simulink model "Controle_v_teta"  (R2018a)
settings: Solver=VariableStepAuto  StartTime=0.0  StopTime=5  RelTol=1e-3
values from neighbouring files (symbols this model uses):
  KDw = 4/(Kw*ts_w)    (= 3.21802091714)    [LineFollower.m]
  KIm = Pm*KPm    (= 0.759312111233)    [LineFollower.m]    (also in malha_fechada.m)
  Km = 455.5    [LineFollower.m]    (also in malha_aberta.m; malha_fechada.m)
  KPm = 4/(Km*ts_m)    (= 0.0585437248445)    [LineFollower.m]    (also in malha_fechada.m)
  KPw = Pw*KDw    (= 80.0965406275)    [LineFollower.m]
  l = 69e-3    (= 0.069)    [LineFollower.m]    (also in malha_aberta.m; malha_fechada.m)
  Pm = 12.97    [LineFollower.m]    (also in malha_aberta.m; malha_fechada.m)
  r = 16e-3    (= 0.016)    [LineFollower.m]    (also in kinematic_model.m; malha_aberta.m; malha_fechada.m)
undefined symbols (not defined in the file or in its folder): KIw
libraries: simulink x3
settings Model: Creator=bruno  LastModifiedBy=bruno

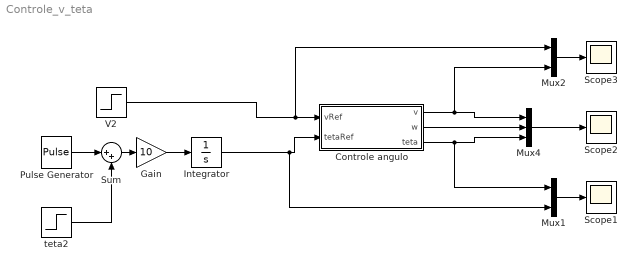
== system Controle_v_teta ==
  Controle angulo : Subsystem
  Gain : Gain  Gain=10
  Integrator : Integrator
  Mux1 : Mux  Inputs=2
  Mux2 : Mux  Inputs=2
  Mux4 : Mux  Inputs=3
  Pulse Generator : DiscretePulseGenerator  PulseType=Time based  PulseWidth=50
  Scope1 : Scope
  Scope2 : Scope
  Scope3 : Scope
  Sum : Sum  Inputs=|++
  V2 : Step  After=2  SampleTime=0
  teta2 : Step  Time=0  After=-0.5  SampleTime=0
  wires:
  V2/1 -> Mux2/1, Controle angulo/1(vRef)
  Mux4/1 -> Scope2/1
  Controle angulo/1(v) -> Mux2/2, Mux4/1
  Controle angulo/2(w) -> Mux4/2
  Controle angulo/3(teta) -> Mux1/1, Mux4/3
  Pulse Generator/1 -> Sum/1
  teta2/1 -> Sum/2
  Sum/1 -> Gain/1
  Mux1/1 -> Scope1/1
  Mux2/1 -> Scope3/1
  Gain/1 -> Integrator/1
  Integrator/1 -> Mux1/2, Controle angulo/2(tetaRef)

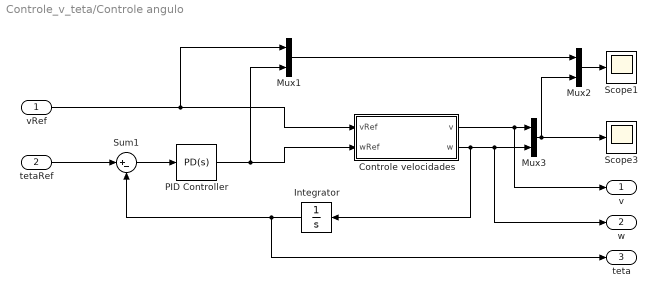
== system Controle_v_teta/Controle angulo ==
  vRef : Inport
  tetaRef : Inport  Port=2
  Controle velocidades : Subsystem
  Integrator : Integrator
  Mux1 : Mux  Inputs=2
  Mux2 : Mux  Inputs=2
  Mux3 : Mux  Inputs=2
  PID Controller : simulink/Continuous/PID Controller  Controller=PD  TimeDomain=Continuous-time  SampleTime=-1  IntegratorMethod=Forward Euler  FilterMethod=Forward Euler  Form=Parallel  UseFilter=on  ControllerParametersSource=internal  P=KPw  I=KIw  D=KDw  N=1  InitialConditionSource=internal  InitialConditionForIntegrator=0  InitialConditionForFilter=0  ExternalReset=none  LimitOutput=off  UpperSaturationLimit=inf  LowerSaturationLimit=-inf  LinearizeAsGain=on  AntiWindupMode=none  Kb=1  TrackingMode=off  Kt=1  PParamMin=[]  PParamMax=[]  IParamMin=[]  IParamMax=[]  DParamMin=[]  DParamMax=[]  NParamMin=[]  NParamMax=[]  KbParamMin=[]  KbParamMax=[]  KtParamMin=[]  KtParamMax=[]  POutMin=[]  POutMax=[]  IOutMin=[]  IOutMax=[]  DOutMin=[]  DOutMax=[]  NOutMin=[]  NOutMax=[]  KbOutMin=[]  KbOutMax=[]  KtOutMin=[]  KtOutMax=[]  IntegratorOutMin=[]  IntegratorOutMax=[]  FilterOutMin=[]  FilterOutMax=[]  SumOutMin=[]  SumOutMax=[]  SumI1OutMin=[]  SumI1OutMax=[]  SumI2OutMin=[]  SumI2OutMax=[]  SumI3OutMin=[]  SumI3OutMax=[]  SumDOutMin=[]  SumDOutMax=[]  SaturationOutMin=[]  SaturationOutMax=[]  IntegratorContinuousStateAttributes=''  IntegratorStateMustResolveToSignalObject=off  IntegratorRTWStateStorageClass=Auto  FilterContinuousStateAttributes=''  FilterStateMustResolveToSignalObject=off  FilterRTWStateStorageClass=Auto  DifferentiatorICPrevScaledInput=0  DifferentiatorOutMin=[]  DifferentiatorOutMax=[]  FilterDiffOutCoefMin=[]  FilterDiffOutCoefMax=[]  SumDenOutMin=[]  SumDenOutMax=[]  SumNumOutMin=[]  SumNumOutMax=[]  ReciprocalOutMin=[]  ReciprocalOutMax=[]  DivideOutMin=[]  DivideOutMax=[]  TunerSelectOption=Transfer Function Based (PID Tuner App)
  Scope1 : Scope
  Scope3 : Scope
  Sum1 : Sum  Inputs=|+-
  v : Outport
  w : Outport  Port=2
  teta : Outport  Port=3
  wires:
  Mux1/1 -> Mux2/1
  Controle velocidades/2(w) -> w/1, Mux3/2, Integrator/1
  Controle velocidades/1(v) -> v/1, Mux3/1
  vRef/1 -> Mux1/1, Controle velocidades/1(vRef)
  PID Controller/1 -> Mux1/2, Controle velocidades/2(wRef)
  Mux2/1 -> Scope1/1
  tetaRef/1 -> Sum1/1
  Mux3/1 -> Mux2/2, Scope3/1
  Integrator/1 -> teta/1, Sum1/2
  Sum1/1 -> PID Controller/1

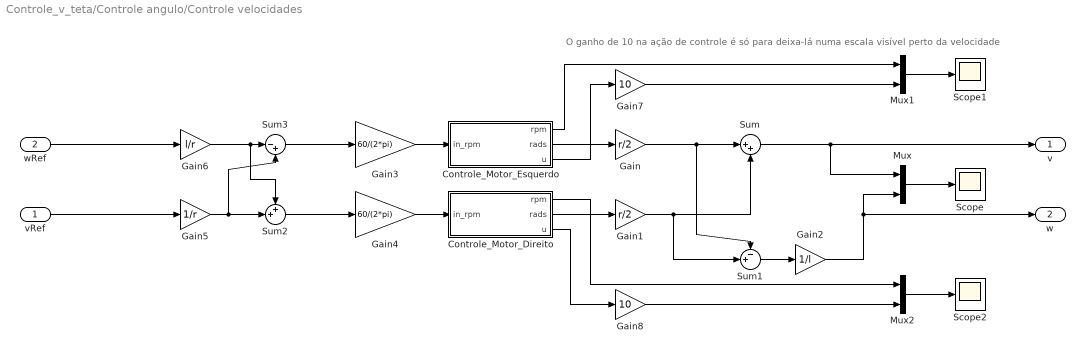
== system Controle_v_teta/Controle angulo/Controle velocidades ==
  note: O ganho de 10 na ação de controle é só para deixa-lá numa escala visível perto da velocidade
  vRef : Inport
  wRef : Inport  Port=2
  Controle_Motor_Direito : Subsystem
  Controle_Motor_Esquerdo : Subsystem
  Gain : Gain  Gain=r/2
  Gain1 : Gain  Gain=r/2
  Gain2 : Gain  Gain=1/l
  Gain3 : Gain  Gain=60/(2*pi)
  Gain4 : Gain  Gain=60/(2*pi)
  Gain5 : Gain  Gain=1/r
  Gain6 : Gain  Gain=l/r
  Gain7 : Gain  Gain=10
  Gain8 : Gain  Gain=10
  Mux : Mux  Inputs=2
  Mux1 : Mux  Inputs=2
  Mux2 : Mux  Inputs=2
  Scope : Scope
  Scope1 : Scope
  Scope2 : Scope
  Sum : Sum  Inputs=|++
  Sum1 : Sum  Inputs=-+|
  Sum2 : Sum  Inputs=++|
  Sum3 : Sum  Inputs=|-+
  v : Outport
  w : Outport  Port=2
  wires:
  Sum2/1 -> Gain4/1
  vRef/1 -> Gain5/1
  Gain7/1 -> Mux1/2
  wRef/1 -> Gain6/1
  Gain2/1 -> w/1, Mux/2
  Gain1/1 -> Sum1/2, Sum/2
  Sum1/1 -> Gain2/1
  Controle_Motor_Direito/2(rads) -> Gain1/1
  Mux2/1 -> Scope2/1
  Gain3/1 -> Controle_Motor_Esquerdo/1(in_rpm)
  Mux/1 -> Scope/1
  Gain4/1 -> Controle_Motor_Direito/1(in_rpm)
  Gain/1 -> Sum1/1, Sum/1
  Gain5/1 -> Sum2/2, Sum3/2
  Mux1/1 -> Scope1/1
  Gain8/1 -> Mux2/2
  Controle_Motor_Esquerdo/3(u) -> Gain7/1
  Gain6/1 -> Sum2/1, Sum3/1
  Sum3/1 -> Gain3/1
  Controle_Motor_Esquerdo/1(rpm) -> Mux1/1
  Controle_Motor_Direito/3(u) -> Gain8/1
  Sum/1 -> v/1, Mux/1
  Controle_Motor_Direito/1(rpm) -> Mux2/1
  Controle_Motor_Esquerdo/2(rads) -> Gain/1

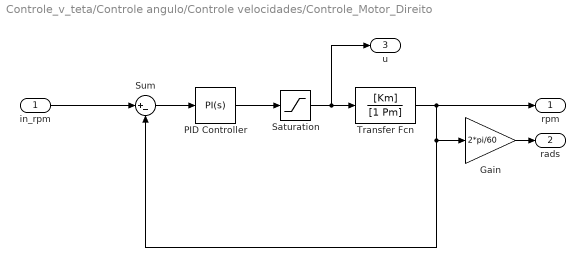
== system Controle_v_teta/Controle angulo/Controle velocidades/Controle_Motor_Direito ==
  in_rpm : Inport
  Gain : Gain  Gain=2*pi/60
  PID Controller : simulink/Continuous/PID Controller  Controller=PI  TimeDomain=Continuous-time  SampleTime=-1  IntegratorMethod=Forward Euler  FilterMethod=Forward Euler  Form=Parallel  UseFilter=on  ControllerParametersSource=internal  P=KPm  I=KIm  D=0  N=0  InitialConditionSource=internal  InitialConditionForIntegrator=0  InitialConditionForFilter=0  ExternalReset=none  LimitOutput=off  UpperSaturationLimit=inf  LowerSaturationLimit=-inf  LinearizeAsGain=on  AntiWindupMode=none  Kb=1  TrackingMode=off  Kt=1  PParamMin=[]  PParamMax=[]  IParamMin=[]  IParamMax=[]  DParamMin=[]  DParamMax=[]  NParamMin=[]  NParamMax=[]  KbParamMin=[]  KbParamMax=[]  KtParamMin=[]  KtParamMax=[]  POutMin=[]  POutMax=[]  IOutMin=[]  IOutMax=[]  DOutMin=[]  DOutMax=[]  NOutMin=[]  NOutMax=[]  KbOutMin=[]  KbOutMax=[]  KtOutMin=[]  KtOutMax=[]  IntegratorOutMin=[]  IntegratorOutMax=[]  FilterOutMin=[]  FilterOutMax=[]  SumOutMin=[]  SumOutMax=[]  SumI1OutMin=[]  SumI1OutMax=[]  SumI2OutMin=[]  SumI2OutMax=[]  SumI3OutMin=[]  SumI3OutMax=[]  SumDOutMin=[]  SumDOutMax=[]  SaturationOutMin=[]  SaturationOutMax=[]  IntegratorContinuousStateAttributes=''  IntegratorStateMustResolveToSignalObject=off  IntegratorRTWStateStorageClass=Auto  FilterContinuousStateAttributes=''  FilterStateMustResolveToSignalObject=off  FilterRTWStateStorageClass=Auto  DifferentiatorICPrevScaledInput=0  DifferentiatorOutMin=[]  DifferentiatorOutMax=[]  FilterDiffOutCoefMin=[]  FilterDiffOutCoefMax=[]  SumDenOutMin=[]  SumDenOutMax=[]  SumNumOutMin=[]  SumNumOutMax=[]  ReciprocalOutMin=[]  ReciprocalOutMax=[]  DivideOutMin=[]  DivideOutMax=[]  TunerSelectOption=Transfer Function Based (PID Tuner App)
  Saturation : Saturate  UpperLimit=100  LowerLimit=-100
  Sum : Sum  Inputs=|+-
  Transfer Fcn : TransferFcn  Numerator=[Km]  Denominator=[1 Pm]
  rpm : Outport
  rads : Outport  Port=2
  u : Outport  Port=3
  wires:
  PID Controller/1 -> Saturation/1
  Transfer Fcn/1 -> rpm/1, Gain/1, Sum/2
  Saturation/1 -> u/1, Transfer Fcn/1
  Sum/1 -> PID Controller/1
  in_rpm/1 -> Sum/1
  Gain/1 -> rads/1

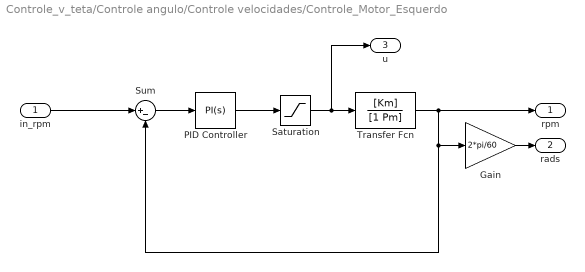
== system Controle_v_teta/Controle angulo/Controle velocidades/Controle_Motor_Esquerdo ==
  in_rpm : Inport
  Gain : Gain  Gain=2*pi/60
  PID Controller : simulink/Continuous/PID Controller  Controller=PI  TimeDomain=Continuous-time  SampleTime=-1  IntegratorMethod=Forward Euler  FilterMethod=Forward Euler  Form=Parallel  UseFilter=on  ControllerParametersSource=internal  P=KPm  I=KIm  D=0  N=0  InitialConditionSource=internal  InitialConditionForIntegrator=0  InitialConditionForFilter=0  ExternalReset=none  LimitOutput=off  UpperSaturationLimit=inf  LowerSaturationLimit=-inf  LinearizeAsGain=on  AntiWindupMode=none  Kb=1  TrackingMode=off  Kt=1  PParamMin=[]  PParamMax=[]  IParamMin=[]  IParamMax=[]  DParamMin=[]  DParamMax=[]  NParamMin=[]  NParamMax=[]  KbParamMin=[]  KbParamMax=[]  KtParamMin=[]  KtParamMax=[]  POutMin=[]  POutMax=[]  IOutMin=[]  IOutMax=[]  DOutMin=[]  DOutMax=[]  NOutMin=[]  NOutMax=[]  KbOutMin=[]  KbOutMax=[]  KtOutMin=[]  KtOutMax=[]  IntegratorOutMin=[]  IntegratorOutMax=[]  FilterOutMin=[]  FilterOutMax=[]  SumOutMin=[]  SumOutMax=[]  SumI1OutMin=[]  SumI1OutMax=[]  SumI2OutMin=[]  SumI2OutMax=[]  SumI3OutMin=[]  SumI3OutMax=[]  SumDOutMin=[]  SumDOutMax=[]  SaturationOutMin=[]  SaturationOutMax=[]  IntegratorContinuousStateAttributes=''  IntegratorStateMustResolveToSignalObject=off  IntegratorRTWStateStorageClass=Auto  FilterContinuousStateAttributes=''  FilterStateMustResolveToSignalObject=off  FilterRTWStateStorageClass=Auto  DifferentiatorICPrevScaledInput=0  DifferentiatorOutMin=[]  DifferentiatorOutMax=[]  FilterDiffOutCoefMin=[]  FilterDiffOutCoefMax=[]  SumDenOutMin=[]  SumDenOutMax=[]  SumNumOutMin=[]  SumNumOutMax=[]  ReciprocalOutMin=[]  ReciprocalOutMax=[]  DivideOutMin=[]  DivideOutMax=[]  TunerSelectOption=Transfer Function Based (PID Tuner App)
  Saturation : Saturate  UpperLimit=100  LowerLimit=-100
  Sum : Sum  Inputs=|+-
  Transfer Fcn : TransferFcn  Numerator=[Km]  Denominator=[1 Pm]
  rpm : Outport
  rads : Outport  Port=2
  u : Outport  Port=3
  wires:
  PID Controller/1 -> Saturation/1
  Saturation/1 -> u/1, Transfer Fcn/1
  Sum/1 -> PID Controller/1
  in_rpm/1 -> Sum/1
  Transfer Fcn/1 -> rpm/1, Gain/1, Sum/2
  Gain/1 -> rads/1
